simulink model "pupillary_relfex"  (R2022a)
settings: Solver=VariableStepAuto  StartTime=0.0  StopTime=10.0  RelTol=1e-3
model workspace: external: MATLAB File C:\Users\bigba\Dropbox\Uni\MSSF\progetti\reflex\pupillary_param.m (data not in the file)
values from neighbouring files (symbols this model uses):
  D = 0.18    [pupillary_param.m]    (also in pupillary_stability.m)
  den = [0.0010000000000000002 0.030000000000000006 0.30000000000000004 1         ]    [pupillary_param.m]    (also in pupillary_stability.m = conv(den,expon_den_pade))
  num = 1    [pupillary_param.m]    (also in pupillary_stability.m = conv(num,expon_num_pade))
settings Model: Creator=bigba  LastModifiedBy=bigba

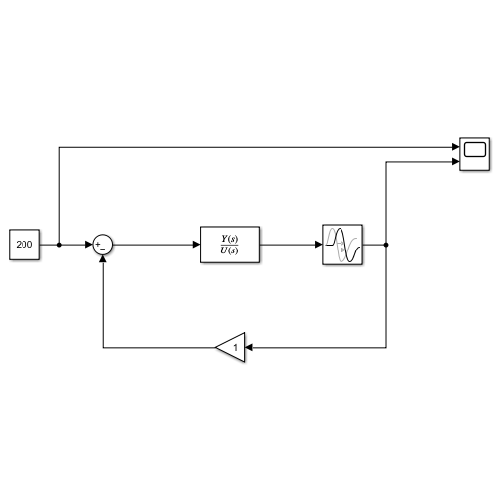
[thumbnail: Simulink's stored preview of the top-level diagram]
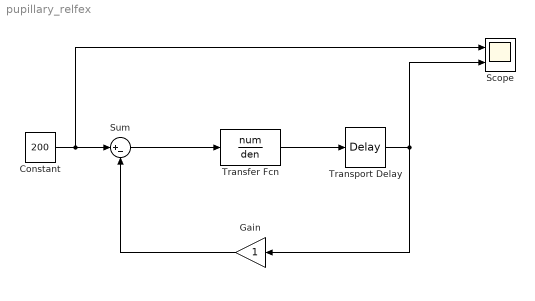
== system pupillary_relfex ==
  Constant : Constant  Value=200
  Gain : Gain
  Scope : Scope  NumInputPorts=2
  Sum : Sum  Inputs=|+-
  Transfer Fcn : TransferFcn  Numerator=num  Denominator=den
  Transport Delay : TransportDelay  DelayTime=D
  wires:
  Constant/1 -> Scope/1, Sum/1
  Sum/1 -> Transfer Fcn/1
  Transfer Fcn/1 -> Transport Delay/1
  Transport Delay/1 -> Gain/1, Scope/2
  Gain/1 -> Sum/2
